simulink model "reorder_test"  (Simulink 8.0)
settings: Solver=ode45  StartTime=0.0  StopTime=1e5+1000  RelTol=1e-3
libraries: xbsIndex_r4 x486, casper_library_delays x4, xps_library x3
(part 1 of 3)
settings Model: Creator=davidm  LastModifiedBy=davidm

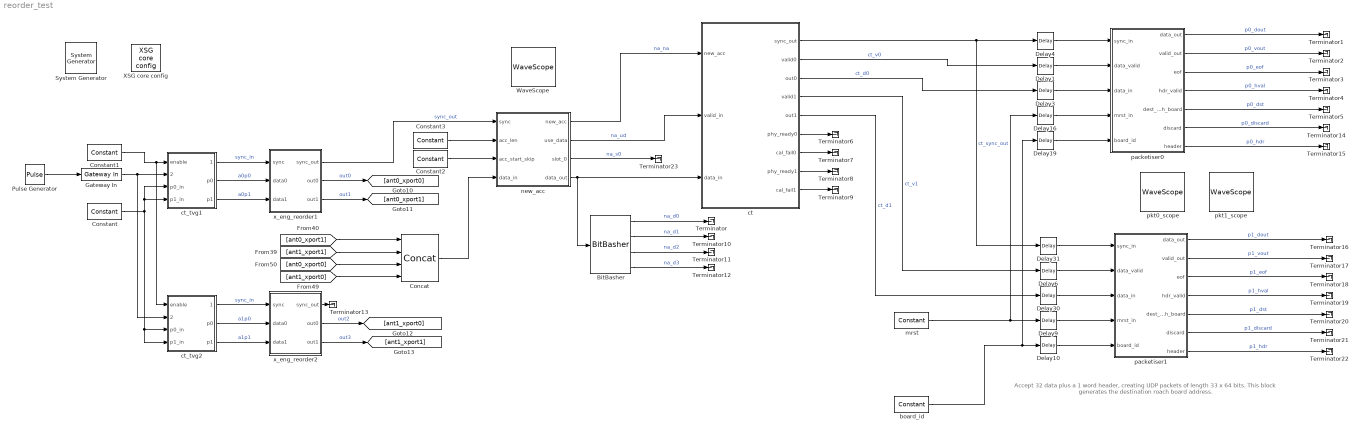
== system reorder_test ==
  note: Accept 32 data plus a 1 word header,
      | creating UDP packets of length 33 x 64 bits.
      | This block generates the destination roach board address.
  " System Generator" : xbsIndex_r4/ System Generator  Tag=genX  xilinxfamily=Kintex7  part=xc7k325t  speed=-3  package=fbg676  synthesis_tool=XST  clock_wrapper=Clock Enables  directory=./netlist  proj_type=Project Navigator  Synth_file=XST Defaults  Impl_file=ISE Defaults  testbench=off  simulink_period=1  sysclk_period=10  dcm_input_clock_period=10  incr_netlist=off  trim_vbits=Everywhere in SubSystem  dbl_ovrd=According to Block Masks  core_generation=According to Block Masks  run_coregen=off  deprecated_control=off  eval_field=0  block_type=sysgen
  BitBasher : xbsIndex_r4/BitBasher  bitexpr=|  display_expr=off  sr_1=1  arith_type1=Unsigned  bin_pt1=0  sr_2=2  arith_type2=Unsigned  bin_pt2=0  sr_3=3  arith_type3=Unsigned  bin_pt3=0  sr_4=4  arith_type4=Unsigned  bin_pt4=0  dbl_ovrd=off  block_type=bitbasher
      | <!DOCTYPE HTML PUBLIC "-//W3C//DTD HTML 4.0//EN" "http://www.w3.org/TR/REC-html40/strict.dtd">
      | <html><head><meta name="qrichtext" content="1" /><style type="text/css">
      | p, li { white-space: pre-wrap; }
      | </style></head><body style=" font-family:'Sans'; font-size:10pt; font-weight:400; font-style:normal;">
      | <p style=" margin-top:12px; margin-bottom:12px; margin-left:0px; margin-right:0px; -qt-block-indent:0; text-indent:0px;"><span style=" font-family:'MS Shell Dlg'; font-size:8pt;">o0={o[63:48]}<br />o1={o[47:32]}<br />o2={o[31:16]}<br />o3={o[15:0]}</span></p></body></html>
  Concat : xbsIndex_r4/Concat  num_inputs=4  dbl_ovrd=off  block_type=concat
  Constant : xbsIndex_r4/Constant  const=hex2dec('dada')  gui_display_data_type=Fixed-point  arith_type=Unsigned  n_bits=16  bin_pt=0  preci_type=Single  exp_width=8  frac_width=24  explicit_period=on  period=1  equ=P=C  opselect=C  inp2=PCIN>>17  opr=+  inp1=P  carry=CIN  dbl_ovrd=off  block_type=constant
  Constant1 : xbsIndex_r4/Constant  const=1  gui_display_data_type=Fixed-point  arith_type=Unsigned  n_bits=1  bin_pt=0  preci_type=Single  exp_width=8  frac_width=24  explicit_period=on  period=1  equ=P=C  opselect=C  inp2=PCIN>>17  opr=+  inp1=P  carry=CIN  dbl_ovrd=off  block_type=constant
  Constant2 : xbsIndex_r4/Constant  const=1  gui_display_data_type=Fixed-point  arith_type=Unsigned  n_bits=16  bin_pt=0  preci_type=Single  exp_width=8  frac_width=24  explicit_period=on  period=1  equ=P=C  opselect=C  inp2=PCIN>>17  opr=+  inp1=P  carry=CIN  dbl_ovrd=off  block_type=constant
  Constant3 : xbsIndex_r4/Constant  const=8  gui_display_data_type=Fixed-point  arith_type=Unsigned  n_bits=16  bin_pt=0  preci_type=Single  exp_width=8  frac_width=24  explicit_period=on  period=1  equ=P=C  opselect=C  inp2=PCIN>>17  opr=+  inp1=P  carry=CIN  dbl_ovrd=off  block_type=constant
  Delay{1,3..4,6,9..10,16,19,30..31} (10 alike) : xbsIndex_r4/Delay  rst=off  infoeditControl=Selection of Reset will increase slice count due to use of real FFs and instead of SRLs  en=off  latency=1  dbl_ovrd=off  reg_retiming=on  block_type=delay
      settings: xl_area=[0, 0, 0, 0, 0, 0, 0]
  Gateway In : xbsIndex_r4/Gateway In  gui_display_data_type=Boolean  arith_type=Boolean  n_bits=16  bin_pt=14  preci_type=Single  exp_width=8  frac_width=24  quantization="Round  (unbiased: +/- Inf)"  overflow=Saturate  period=1  dbl_ovrd=off  timing_constraint=None  locs_specified=off  LOCs={}  UseAsADC=off  ADCChannel='1'  inherit_from_input=off  hdl_port=on  block_type=gatewayin
  Pulse Generator : DiscretePulseGenerator  Period=1e9  PhaseDelay=2
  Terminator{,1..23} (24 alike) : Terminator
  WaveScope : xbsIndex_r4/WaveScope  block_type=wavescope
  XSG core config : xps_library/XSG core config  Tag=xps:xsg  hw_sys=ROACH2:sx475t  clk_src=sys_clk  ROACH_clk_src=sys_clk  ROACH2_clk_src=sys_clk  MKDIG_clk_src=sys_clk  clk_rate=100  sample_period=1  synthesis_tool=XST
  board_id : xbsIndex_r4/Constant  const=0  gui_display_data_type=Fixed-point  arith_type=Unsigned  n_bits=4  bin_pt=0  preci_type=Single  exp_width=8  frac_width=24  explicit_period=on  period=1  equ=P=C  opselect=C  inp2=PCIN>>17  opr=+  inp1=P  carry=CIN  dbl_ovrd=off  block_type=constant
  ct : Subsystem  mask{freq_chan=12, x_acc_len=3, bram_latency=2, ip_bits=16}
      mask prompts: freq_chan "No. of frequency channels (2 ^ ?)"; x_acc_len "X-eng Accumulation length (2^? samples):"; bram_latency "bram latency"; ip_bits "Input channel bitwidth"
  ct_tvg1 : Subsystem  mask{num_channels_bits=12, channel_bits=8, ant=0}
      mask prompts: num_channels_bits "Number of channels (2^?):"; channel_bits "Bits per channel:"; ant "Antenna # [0, 15]"
  ct_tvg2 : Subsystem  mask{num_channels_bits=12, channel_bits=8, ant=1}
      mask prompts: num_channels_bits "Number of channels (2^?):"; channel_bits "Bits per channel:"; ant "Antenna # [0, 15]"
  mrst : xbsIndex_r4/Constant  const=0  gui_display_data_type=Boolean  arith_type=Boolean  n_bits=4  bin_pt=0  preci_type=Single  exp_width=8  frac_width=24  explicit_period=on  period=1  equ=P=C  opselect=C  inp2=PCIN>>17  opr=+  inp1=P  carry=CIN  dbl_ovrd=off  block_type=constant
  new_acc : Subsystem
  packetiser0 : Subsystem  mask{payload_bits=1, n_x_board=2, freq_chan=12, n_boards=1, gbe_port=0}
      mask prompts: payload_bits "Payload length in 64bit words (2^?)"; n_x_board "Number of x-engines per ROACH board (2^?)"; freq_chan "Number of frequencies (2^?)"; n_boards "Number of  ROACH boards (2 ^ ?)"; gbe_port "Port # (0 or 1)"
      mask help: Package 32 bit data into 64 bits and identify data as coming from antenna 0 or 1
      mask init:
      | n_x = n_x_board - 1;
  packetiser1 : Subsystem  mask{payload_bits=1, n_x_board=2, freq_chan=12, n_boards=1, gbe_port=1}
      mask prompts: payload_bits "Payload length in 64bit words (2^?)"; n_x_board "Number of x-engines per ROACH board (2^?)"; freq_chan "Number of frequencies (2^?)"; n_boards "Number of  ROACH boards (2 ^ ?)"; gbe_port "Port # (0 or 1)"
      mask help: Package 32 bit data into 64 bits and identify data as coming from antenna 0 or 1
      mask init:
      | n_x = n_x_board - 1;
  pkt0_scope : xbsIndex_r4/WaveScope  block_type=wavescope
  pkt1_scope : xbsIndex_r4/WaveScope  block_type=wavescope
  x_eng_reorder1 : Subsystem  mask{freq_chan=12, num_data_bits=16, bram_latency=2, n_boards=1, n_x_board=2}
      mask prompts: freq_chan "Number of Frequency Channels (2 ^ ?)"; num_data_bits "Incomin data width in bits"; bram_latency "BRAM Latency"; n_boards "Number of ROACH boards (2 ^ ?)"; n_x_board "Number of X-engines per ROACH board (2 ^ ?)"
      mask help:
      | Reorders channels for transmission to X-engines in two stages.
      |
      | In the first stage, total of P channels on both inputs (P/2 on each input)
      | are reordered as follows:
      |
      | Input data0 has channels: 0, 2, 4, ..., P-2.
      | Input data1 has channels: 1, 3, 5, ..., P-1.
      | Then,
      | Output out0 has channels: 0, 1, 2, ..., P/2 -1.
      | Output out1 has channels: P/2, P/2 + 1, ..., P-1.
      |
      | Here P = 2 ^ (N - B),
      | where 2 ^ N = no. of total frequency channels
      | and 2 ^ B = total number of ROACH boards
      |
      | In the second stage, the channels on the each output are reordered in a way
      | that when presented to the 10 GbE port, they appear in the following order:
      | First channel to the first X-engine connected to the receiving 10gbE port of all ROACH boards.
      | First channel to the second X-engine connected to the receiving 10GbE port of all ROACH boards.
      | and so on.
      mask init:
      | n_x = n_x_board - 1;
  x_eng_reorder2 : Subsystem  mask{freq_chan=12, num_data_bits=16, bram_latency=2, n_boards=1, n_x_board=2}
      mask prompts: freq_chan "Number of Frequency Channels (2 ^ ?)"; num_data_bits "Incomin data width in bits"; bram_latency "BRAM Latency"; n_boards "Number of ROACH boards (2 ^ ?)"; n_x_board "Number of X-engines per ROACH board (2 ^ ?)"
      mask help:
      | Reorders channels for transmission to X-engines in two stages.
      |
      | In the first stage, total of P channels on both inputs (P/2 on each input)
      | are reordered as follows:
      |
      | Input data0 has channels: 0, 2, 4, ..., P-2.
      | Input data1 has channels: 1, 3, 5, ..., P-1.
      | Then,
      | Output out0 has channels: 0, 1, 2, ..., P/2 -1.
      | Output out1 has channels: P/2, P/2 + 1, ..., P-1.
      |
      | Here P = 2 ^ (N - B),
      | where 2 ^ N = no. of total frequency channels
      | and 2 ^ B = total number of ROACH boards
      |
      | In the second stage, the channels on the each output are reordered in a way
      | that when presented to the 10 GbE port, they appear in the following order:
      | First channel to the first X-engine connected to the receiving 10gbE port of all ROACH boards.
      | First channel to the second X-engine connected to the receiving 10GbE port of all ROACH boards.
      | and so on.
      mask init:
      | n_x = n_x_board - 1;
  wires:
  ct_tvg1/1(sync_out) -> x_eng_reorder1/1(sync)  "sync_in"
  ct_tvg1/2(p0) -> x_eng_reorder1/2(data0)  "a0p0"
  ct_tvg1/3(p1) -> x_eng_reorder1/3(data1)  "a0p1"
  Pulse Generator/1 -> Gateway In/1
  Gateway In/1 -> ct_tvg2/2(sync_in), ct_tvg1/2(sync_in)
  Constant/1 -> ct_tvg2/4(p1_in), ct_tvg2/3(p0_in), ct_tvg1/4(p1_in), ct_tvg1/3(p0_in)
  Constant1/1 -> ct_tvg2/1(enable), ct_tvg1/1(enable)
  x_eng_reorder1/1(sync_out) -> new_acc/1(sync)  "sync_out"
  x_eng_reorder1/2(out0) -> [ant0_xport0]  "out0"
  x_eng_reorder1/3(out1) -> [ant0_xport1]  "out1"
  Constant2/1 -> new_acc/3(acc_start_skip)
  Constant3/1 -> new_acc/2(acc_len)
  new_acc/1(new_acc) -> ct/1(new_acc)  "na_na"
  new_acc/2(use_data) -> ct/2(valid_in)  "na_ud"
  new_acc/4(data_out) -> BitBasher/1, ct/3(data_in)
  ct/1(sync_out) -> Delay4/1, Delay31/1  "ct_sync_out"
  ct/2(valid0) -> Delay1/1  "ct_v0"
  ct/3(out0) -> Delay3/1  "ct_d0"
  ct/4(valid1) -> Delay6/1  "ct_v1"
  ct/5(out1) -> Delay30/1  "ct_d1"
  ct/6(phy_ready0) -> Terminator6/1
  ct/7(cal_fail0) -> Terminator7/1
  ct/8(phy_ready1) -> Terminator8/1
  ct/9(cal_fail1) -> Terminator9/1
  ct_tvg2/1(sync_out) -> x_eng_reorder2/1(sync)  "sync_in"
  ct_tvg2/2(p0) -> x_eng_reorder2/2(data0)  "a1p0"
  ct_tvg2/3(p1) -> x_eng_reorder2/3(data1)  "a1p1"
  x_eng_reorder2/2(out0) -> [ant1_xport0]  "out2"
  x_eng_reorder2/3(out1) -> [ant1_xport1]  "out3"
  Concat/1 -> new_acc/4(data_in)
  BitBasher/1 -> Terminator/1  "na_d0"
  BitBasher/2 -> Terminator10/1  "na_d1"
  BitBasher/3 -> Terminator11/1  "na_d2"
  BitBasher/4 -> Terminator12/1  "na_d3"
  x_eng_reorder2/1(sync_out) -> Terminator13/1
  Delay4/1 -> packetiser0/1(sync_in)
  Delay1/1 -> packetiser0/2(data_valid)
  Delay3/1 -> packetiser0/3(data_in)
  Delay16/1 -> packetiser0/4(mrst_in)
  Delay19/1 -> packetiser0/5(board_id)
  Delay31/1 -> packetiser1/1(sync_in)
  Delay6/1 -> packetiser1/2(data_valid)
  Delay30/1 -> packetiser1/3(data_in)
  Delay9/1 -> packetiser1/4(mrst_in)
  Delay10/1 -> packetiser1/5(board_id)
  board_id/1 -> Delay19/1, Delay10/1
  mrst/1 -> Delay16/1, Delay9/1
  packetiser0/1(data_out) -> Terminator1/1  "p0_dout"
  packetiser0/2(valid_out) -> Terminator2/1  "p0_vout"
  packetiser0/3(eof) -> Terminator3/1  "p0_eof"
  packetiser0/4(hdr_valid) -> Terminator4/1  "p0_hval"
  packetiser0/5(dest_roach_board) -> Terminator5/1  "p0_dst"
  packetiser0/6(discard) -> Terminator14/1  "p0_discard"
  packetiser0/7(header) -> Terminator15/1  "p0_hdr"
  packetiser1/1(data_out) -> Terminator16/1  "p1_dout"
  packetiser1/2(valid_out) -> Terminator17/1  "p1_vout"
  packetiser1/3(eof) -> Terminator18/1  "p1_eof"
  packetiser1/4(hdr_valid) -> Terminator19/1  "p1_hval"
  packetiser1/5(dest_roach_board) -> Terminator20/1  "p1_dst"
  packetiser1/6(discard) -> Terminator21/1  "p1_discard"
  packetiser1/7(header) -> Terminator22/1  "p1_hdr"
  [ant0_xport1] -> Concat/1
  [ant1_xport1] -> Concat/2
  [ant0_xport0] -> Concat/3
  [ant1_xport0] -> Concat/4
  new_acc/3(slot_0) -> Terminator23/1  "na_s0"

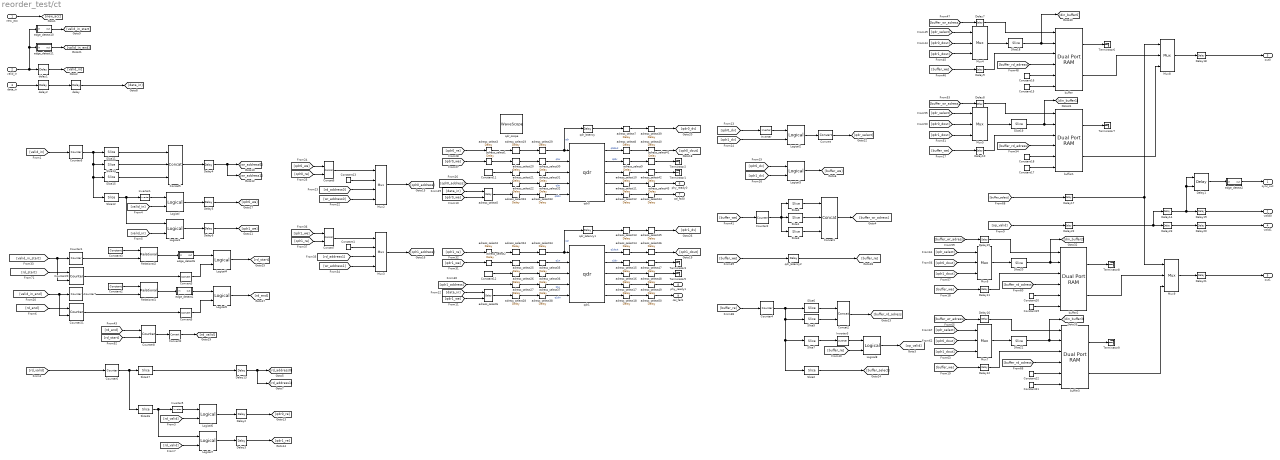
== system reorder_test/ct ==
  new_acc : Inport
  valid_in : Inport  Port=2
  data_in : Inport  Port=3
  Concat1 : xbsIndex_r4/Concat  num_inputs=3  dbl_ovrd=off  block_type=concat
  Concat2 : xbsIndex_r4/Concat  num_inputs=2  dbl_ovrd=off  block_type=concat
  Concat5 : xbsIndex_r4/Concat  num_inputs=3  dbl_ovrd=off  block_type=concat
  Concat6 : xbsIndex_r4/Concat  num_inputs=2  dbl_ovrd=off  block_type=concat
  Concat7 : xbsIndex_r4/Concat  num_inputs=2  dbl_ovrd=off  block_type=concat
  Constant1 : xbsIndex_r4/Constant  const=0  gui_display_data_type=Fixed-point  arith_type=Unsigned  n_bits=freq_chan + x_acc_len - 1  bin_pt=0  preci_type=Single  exp_width=8  frac_width=24  explicit_period=on  period=1  equ=P=C  opselect=C  inp2=PCIN>>17  opr=+  inp1=P  carry=CIN  dbl_ovrd=off  block_type=constant
      settings: block_version=11.4
  Constant11 : xbsIndex_r4/Constant  const=255  gui_display_data_type=Fixed-point  arith_type=Unsigned  n_bits=8  bin_pt=0  preci_type=Single  exp_width=8  frac_width=24  explicit_period=on  period=1  equ=P=C  opselect=C  inp2=PCIN>>17  opr=+  inp1=P  carry=CIN  dbl_ovrd=off  block_type=constant
  Constant12 : xbsIndex_r4/Constant  const=255  gui_display_data_type=Fixed-point  arith_type=Unsigned  n_bits=8  bin_pt=0  preci_type=Single  exp_width=8  frac_width=24  explicit_period=on  period=1  equ=P=C  opselect=C  inp2=PCIN>>17  opr=+  inp1=P  carry=CIN  dbl_ovrd=off  block_type=constant
  Constant13 : xbsIndex_r4/Constant  const=0  gui_display_data_type=Fixed-point  arith_type=Unsigned  n_bits=freq_chan + x_acc_len - 1  bin_pt=0  preci_type=Single  exp_width=8  frac_width=24  explicit_period=on  period=1  equ=P=C  opselect=C  inp2=PCIN>>17  opr=+  inp1=P  carry=CIN  dbl_ovrd=off  block_type=constant
      settings: block_version=11.4
  Constant{15,17,19,21} (4 alike) : xbsIndex_r4/Constant  const=0  gui_display_data_type=Fixed-point  arith_type=Boolean  n_bits=16  bin_pt=14  preci_type=Single  exp_width=8  frac_width=24  explicit_period=on  period=1  equ=P=C  opselect=C  inp2=PCIN>>17  opr=+  inp1=P  carry=CIN  dbl_ovrd=off  block_type=constant
      settings: block_version=11.4
  Constant{16,18,20,22} (4 alike) : xbsIndex_r4/Constant  const=0  gui_display_data_type=Fixed-point  arith_type=Unsigned  n_bits=64  bin_pt=0  preci_type=Single  exp_width=8  frac_width=24  explicit_period=on  period=1  equ=P=C  opselect=C  inp2=PCIN>>17  opr=+  inp1=P  carry=CIN  dbl_ovrd=off  block_type=constant
      settings: block_version=11.4
  Constant2 : xbsIndex_r4/Constant  const=2 ^ (freq_chan + x_acc_len - 1) - 3  gui_display_data_type=Fixed-point  arith_type=Unsigned  n_bits=freq_chan + x_acc_len - 1  bin_pt=0  preci_type=Single  exp_width=8  frac_width=24  explicit_period=on  period=1  equ=P=C  opselect=C  inp2=PCIN>>17  opr=+  inp1=P  carry=CIN  dbl_ovrd=off  block_type=constant
      settings: block_version=11.4
  Constant3 : xbsIndex_r4/Constant  const=2 ^ (freq_chan + x_acc_len - 1) - 3  gui_display_data_type=Fixed-point  arith_type=Unsigned  n_bits=freq_chan + x_acc_len - 1  bin_pt=0  preci_type=Single  exp_width=8  frac_width=24  explicit_period=on  period=1  equ=P=C  opselect=C  inp2=PCIN>>17  opr=+  inp1=P  carry=CIN  dbl_ovrd=off  block_type=constant
      settings: block_version=11.4
  Convert : xbsIndex_r4/Convert  gui_display_data_type=Fixed-point  arith_type=Unsigned  n_bits=1  bin_pt=0  float_type=Single  exp_bits=8  fraction_bits=24  quantization=Truncate  overflow=Wrap  en=off  latency=0  dbl_ovrd=off  pipeline=off  block_type=convert
      settings: block_version=11.4
  Convert2 : xbsIndex_r4/Convert  gui_display_data_type=Fixed-point  arith_type=Boolean  n_bits=16  bin_pt=14  float_type=Single  exp_bits=8  fraction_bits=24  quantization=Truncate  overflow=Wrap  en=off  latency=0  dbl_ovrd=off  pipeline=off  block_type=convert
      settings: block_version=11.4
  Convert3 : xbsIndex_r4/Convert  gui_display_data_type=Fixed-point  arith_type=Boolean  n_bits=16  bin_pt=14  float_type=Single  exp_bits=8  fraction_bits=24  quantization=Truncate  overflow=Wrap  en=off  latency=0  dbl_ovrd=off  pipeline=off  block_type=convert
      settings: block_version=11.4
  Convert5 : xbsIndex_r4/Convert  gui_display_data_type=Fixed-point  arith_type=Boolean  n_bits=16  bin_pt=14  float_type=Single  exp_bits=8  fraction_bits=24  quantization=Truncate  overflow=Wrap  en=off  latency=0  dbl_ovrd=off  pipeline=off  block_type=convert
      settings: block_version=11.4
  Counter1 : xbsIndex_r4/Counter  cnt_type=Free Running  cnt_to=10  operation=Up  start_count=0  cnt_by_val=1  arith_type=Unsigned  n_bits=freq_chan + x_acc_len - 1  bin_pt=0  load_pin=off  rst=on  en=off  explicit_period=off  period=1  dbl_ovrd=off  use_behavioral_HDL=off  implementation=Fabric  block_type=counter
      settings: block_version=11.4
  Counter2 : xbsIndex_r4/Counter  cnt_type=Free Running  cnt_to=10  operation=Up  start_count=0  cnt_by_val=1  arith_type=Unsigned  n_bits=x_acc_len + 2  bin_pt=0  load_pin=off  rst=off  en=on  explicit_period=off  period=1  dbl_ovrd=off  use_behavioral_HDL=off  implementation=Fabric  block_type=counter
      settings: block_version=11.4
  Counter20 : xbsIndex_r4/Counter  cnt_type=Free Running  cnt_to=10  operation=Up  start_count=0  cnt_by_val=1  arith_type=Unsigned  n_bits=1  bin_pt=0  load_pin=off  rst=on  en=on  explicit_period=off  period=1  dbl_ovrd=off  use_behavioral_HDL=off  implementation=Fabric  block_type=counter
      settings: block_version=11.4
  Counter21 : xbsIndex_r4/Counter  cnt_type=Free Running  cnt_to=10  operation=Up  start_count=0  cnt_by_val=1  arith_type=Unsigned  n_bits=1  bin_pt=0  load_pin=off  rst=on  en=on  explicit_period=off  period=1  dbl_ovrd=off  use_behavioral_HDL=off  implementation=Fabric  block_type=counter
      settings: block_version=11.4
  Counter4 : xbsIndex_r4/Counter  cnt_type=Free Running  cnt_to=10  operation=Up  start_count=0  cnt_by_val=1  arith_type=Unsigned  n_bits=x_acc_len + 2  bin_pt=0  load_pin=off  rst=off  en=on  explicit_period=off  period=1  dbl_ovrd=off  use_behavioral_HDL=off  implementation=Fabric  block_type=counter
      settings: block_version=11.4
  Counter5 : xbsIndex_r4/Counter  cnt_type=Free Running  cnt_to=10  operation=Up  start_count=0  cnt_by_val=1  arith_type=Unsigned  n_bits=freq_chan + x_acc_len  bin_pt=0  load_pin=off  rst=off  en=on  explicit_period=off  period=1  dbl_ovrd=off  use_behavioral_HDL=off  implementation=Fabric  block_type=counter
      settings: block_version=11.4
  Counter6 : xbsIndex_r4/Counter  cnt_type=Free Running  cnt_to=10  operation=Up  start_count=0  cnt_by_val=1  arith_type=Unsigned  n_bits=freq_chan + x_acc_len  bin_pt=0  load_pin=off  rst=off  en=on  explicit_period=off  period=1  dbl_ovrd=off  use_behavioral_HDL=off  implementation=Fabric  block_type=counter
      settings: block_version=11.4
  Counter7 : xbsIndex_r4/Counter  cnt_type=Free Running  cnt_to=10  operation=Up  start_count=0  cnt_by_val=1  arith_type=Unsigned  n_bits=freq_chan + x_acc_len - 1  bin_pt=0  load_pin=off  rst=on  en=off  explicit_period=off  period=1  dbl_ovrd=off  use_behavioral_HDL=off  implementation=Fabric  block_type=counter
      settings: block_version=11.4
  Counter8 : xbsIndex_r4/Counter  cnt_type=Free Running  cnt_to=10  operation=Up  start_count=0  cnt_by_val=1  arith_type=Unsigned  n_bits=1  bin_pt=0  load_pin=off  rst=on  en=on  explicit_period=off  period=1  dbl_ovrd=off  use_behavioral_HDL=off  implementation=Fabric  block_type=counter
      settings: block_version=11.4
  Delay1 : xbsIndex_r4/Delay  rst=off  infoeditControl=Selection of Reset will increase slice count due to use of real FFs and instead of SRLs  en=on  latency=1  dbl_ovrd=off  reg_retiming=on  block_type=delay
      settings: block_version=11.4
  Delay{2..16,23} (16 alike) : xbsIndex_r4/Delay  rst=off  infoeditControl=Selection of Reset will increase slice count due to use of real FFs and instead of SRLs  en=off  latency=1  dbl_ovrd=off  reg_retiming=on  block_type=delay
      settings: block_version=11.4
  Delay17 : xbsIndex_r4/Delay  rst=off  infoeditControl=Selection of Reset will increase slice count due to use of real FFs and instead of SRLs  en=off  latency=bram_latency  dbl_ovrd=off  reg_retiming=on  block_type=delay
      settings: block_version=11.4
  Delay{18..21} (4 alike) : xbsIndex_r4/Delay  rst=off  infoeditControl=Selection of Reset will increase slice count due to use of real FFs and instead of SRLs  en=off  latency=2  dbl_ovrd=off  reg_retiming=on  block_type=delay
      settings: block_version=11.4
  Delay22 : xbsIndex_r4/Delay  rst=off  infoeditControl=Selection of Reset will increase slice count due to use of real FFs and instead of SRLs  en=off  latency=bram_latency  dbl_ovrd=off  reg_retiming=on  block_type=delay
      settings: block_version=11.4
  Inverter{,1,3,5} (4 alike) : xbsIndex_r4/Inverter  en=off  latency=0  dbl_ovrd=off  block_type=inv
      settings: block_version=11.4
  Logical{,1..2,4..8} (8 alike) : xbsIndex_r4/Logical  logical_function=AND  inputs=2  en=off  latency=0  precision=Full  arith_type=Unsigned  n_bits=16  bin_pt=0  align_bp=on  dbl_ovrd=off  block_type=logical
      settings: block_version=11.4
  Logical3 : xbsIndex_r4/Logical  logical_function=XOR  inputs=2  en=off  latency=0  precision=Full  arith_type=Unsigned  n_bits=16  bin_pt=0  align_bp=on  dbl_ovrd=off  block_type=logical
      settings: block_version=11.4
  Mux2 : xbsIndex_r4/Mux  inputs=3  en=off  latency=1  precision=Full  arith_type=Unsigned  n_bits=16  bin_pt=14  quantization=Truncate  overflow=Wrap  dbl_ovrd=off  block_type=mux
      settings: block_version=11.4
  Mux3 : xbsIndex_r4/Mux  inputs=3  en=off  latency=1  precision=Full  arith_type=Unsigned  n_bits=16  bin_pt=14  quantization=Truncate  overflow=Wrap  dbl_ovrd=off  block_type=mux
      settings: block_version=11.4
  Mux{4..9} (6 alike) : xbsIndex_r4/Mux  inputs=2  en=off  latency=1  precision=Full  arith_type=Unsigned  n_bits=16  bin_pt=14  quantization=Truncate  overflow=Wrap  dbl_ovrd=off  block_type=mux
      settings: block_version=11.4
  Relational1 : xbsIndex_r4/Relational  mode=a=b  en=off  latency=1  dbl_ovrd=off  block_type=relational
  Relational2 : xbsIndex_r4/Relational  mode=a=b  en=off  latency=1  dbl_ovrd=off  block_type=relational
  Slice1 : xbsIndex_r4/Slice  nbits=1  boolean_output=off  mode=Lower Bit Location + Width  bit1=0  base1=MSB of Input  bit0=0  base0=LSB of Input  dbl_ovrd=off  block_type=slice
      settings: block_version=10.1.3
  Slice11 : xbsIndex_r4/Slice  nbits=1  boolean_output=off  mode=Upper Bit Location + Width  bit1=0  base1=MSB of Input  bit0=1  base0=LSB of Input  dbl_ovrd=off  block_type=slice
      settings: block_version=10.1.3
  Slice12 : xbsIndex_r4/Slice  nbits=1  boolean_output=on  mode=Lower Bit Location + Width  bit1=0  base1=MSB of Input  bit0=0  base0=LSB of Input  dbl_ovrd=off  block_type=slice
      settings: block_version=10.1.3
  Slice14 : xbsIndex_r4/Slice  nbits=freq_chan - 2  boolean_output=off  mode=Lower Bit Location + Width  bit1=0  base1=MSB of Input  bit0=1  base0=LSB of Input  dbl_ovrd=off  block_type=slice
      settings: block_version=10.1.3
  Slice15 : xbsIndex_r4/Slice  nbits=x_acc_len  boolean_output=off  mode=Lower Bit Location + Width  bit1=0  base1=MSB of Input  bit0=freq_chan - 1  base0=LSB of Input  dbl_ovrd=off  block_type=slice
      settings: block_version=10.1.3
  Slice16 : xbsIndex_r4/Slice  nbits=1  boolean_output=on  mode=Lower Bit Location + Width  bit1=0  base1=MSB of Input  bit0=0  base0=LSB of Input  dbl_ovrd=off  block_type=slice
      settings: block_version=10.1.3
  Slice17 : xbsIndex_r4/Slice  nbits=freq_chan + x_acc_len - 1  boolean_output=off  mode=Lower Bit Location + Width  bit1=0  base1=MSB of Input  bit0=1  base0=LSB of Input  dbl_ovrd=off  block_type=slice
      settings: block_version=10.1.3
  Slice18 : xbsIndex_r4/Slice  nbits=ip_bits  boolean_output=off  mode=Lower Bit Location + Width  bit1=0  base1=MSB of Input  bit0=ip_bits * 3  base0=LSB of Input  dbl_ovrd=off  block_type=slice
      settings: block_version=10.1.3
  Slice19 : xbsIndex_r4/Slice  nbits=ip_bits  boolean_output=off  mode=Lower Bit Location + Width  bit1=0  base1=MSB of Input  bit0=ip_bits * 2  base0=LSB of Input  dbl_ovrd=off  block_type=slice
      settings: block_version=10.1.3
  Slice2 : xbsIndex_r4/Slice  nbits=1  boolean_output=off  mode=Lower Bit Location + Width  bit1=0  base1=MSB of Input  bit0=x_acc_len - 1  base0=LSB of Input  dbl_ovrd=off  block_type=slice
      settings: block_version=10.1.3
  Slice20 : xbsIndex_r4/Slice  nbits=ip_bits  boolean_output=off  mode=Lower Bit Location + Width  bit1=0  base1=MSB of Input  bit0=ip_bits  base0=LSB of Input  dbl_ovrd=off  block_type=slice
      settings: block_version=10.1.3
  Slice21 : xbsIndex_r4/Slice  nbits=ip_bits  boolean_output=off  mode=Lower Bit Location + Width  bit1=0  base1=MSB of Input  bit0=0  base0=LSB of Input  dbl_ovrd=off  block_type=slice
      settings: block_version=10.1.3
  Slice3 : xbsIndex_r4/Slice  nbits=x_acc_len  boolean_output=off  mode=Lower Bit Location + Width  bit1=0  base1=MSB of Input  bit0=1  base0=LSB of Input  dbl_ovrd=off  block_type=slice
      settings: block_version=10.1.3
  Slice4 : xbsIndex_r4/Slice  nbits=1  boolean_output=on  mode=Upper Bit Location + Width  bit1=0  base1=MSB of Input  bit0=0  base0=LSB of Input  dbl_ovrd=off  block_type=slice
      settings: block_version=10.1.3
  Slice5 : xbsIndex_r4/Slice  nbits=x_acc_len - 2  boolean_output=off  mode=Lower Bit Location + Width  bit1=0  base1=MSB of Input  bit0=0  base0=LSB of Input  dbl_ovrd=off  block_type=slice
      settings: block_version=10.1.3
  Slice6 : xbsIndex_r4/Slice  nbits=2  boolean_output=off  mode=Upper Bit Location + Width  bit1=0  base1=MSB of Input  bit0=0  base0=LSB of Input  dbl_ovrd=off  block_type=slice
      settings: block_version=10.1.3
  Slice7 : xbsIndex_r4/Slice  nbits=1  boolean_output=on  mode=Lower Bit Location + Width  bit1=0  base1=MSB of Input  bit0=x_acc_len - 2  base0=LSB of Input  dbl_ovrd=off  block_type=slice
      settings: block_version=10.1.3
  Terminator{1..3,5..9} (8 alike) : Terminator
  adress_select{1..4,7..50} (48 alike) : xbsIndex_r4/Delay  rst=off  infoeditControl=Selection of Reset will increase slice count due to use of real FFs and instead of SRLs  en=off  latency=1  dbl_ovrd=off  reg_retiming=on  block_type=delay
      settings: block_version=11.4
  adress_select5 : xbsIndex_r4/Delay  rst=off  infoeditControl=Selection of Reset will increase slice count due to use of real FFs and instead of SRLs  en=on  latency=1  dbl_ovrd=off  reg_retiming=on  block_type=delay
      settings: block_version=11.4
  adress_select6 : xbsIndex_r4/Delay  rst=off  infoeditControl=Selection of Reset will increase slice count due to use of real FFs and instead of SRLs  en=on  latency=1  dbl_ovrd=off  reg_retiming=on  block_type=delay
      settings: block_version=11.4
  buffer{,1..3} (4 alike) : xbsIndex_r4/Dual Port RAM  depth=2 ^ (x_acc_len + 2)  initVector=0  distributed_mem=Block RAM  init_a=0  init_b=0  rst_a=off  rst_b=off  en_a=off  en_b=off  latency=bram_latency  write_mode_A=Read Before Write  write_mode_B=Read Before Write  dbl_ovrd=off  optimize=Area  block_type=dpram
      settings: block_version=11.4
  delay : xbsIndex_r4/Delay  rst=off  infoeditControl=Selection of Reset will increase slice count due to use of real FFs and instead of SRLs  en=off  latency=1  dbl_ovrd=off  reg_retiming=on  block_type=delay
      settings: block_version=11.4
  delay1 : xbsIndex_r4/Delay  rst=off  infoeditControl=Selection of Reset will increase slice count due to use of real FFs and instead of SRLs  en=off  latency=1  dbl_ovrd=off  reg_retiming=on  block_type=delay
      settings: block_version=11.4
  delay2 : xbsIndex_r4/Delay  rst=off  infoeditControl=Selection of Reset will increase slice count due to use of real FFs and instead of SRLs  en=off  latency=1  dbl_ovrd=off  reg_retiming=on  block_type=delay
      settings: block_version=11.4
  edge_detect1 : Subsystem  AncestorBlock=casper_library_misc/edge_detect  mask(edge_detect){edge=Rising, polarity=Active High, x_in=[0 0.08 0.08 0.16 0.16 0.24 0.24 0.32 0.32 0.4], y_in=[-1 -1  1  1  1  1  1  1  1  1], x_out=[0.6 0.68 0.68 0.76 0.76 0.84 0.84 0.92 0.92 1], y_out=[-1 -1  1  1 -1 -1 -1 -1 -1 -1]}
      mask prompts: edge "Edge Type"; polarity "Output Polarity"; x_in "Input X Positions"; y_in "Input Y Positions"; x_out "Output X Positions"; y_out "Output Y Positions"
      mask help: Output is active for one-cycle after each edge of the specified type (i.e. rising, falling or both).
      mask init:
      | edge_detect_init(gcb,...
      |     'edge',edge,...
      |     'polarity',polarity,...
      |     'x_in',x_in,...
      |     'x_out',x_out,...
      |     'y_in',y_in,...
      |     'y_out',y_out);
      | 
      | x_in_num=str2num(getfield(getfield(get_param(gcb,'UserData'),'parameters'),'x_in'));
      | x_out_num=str2num(getfield(getfield(get_param(gcb,'UserData'),'parameters'),'x_out'));
      | y_in_num=str2num(getfield(getfield(get_param(gcb,'UserData'),'parameters'),'y_in'));
      | y_out_num=str2num(getfield(getfield(get_param(gcb,'UserData'),'parameters'),'y_out'));
      settings: AttributesFormatString=|
      | rising edges
      | active high
      mask Help: Output is active for one-cycle after each edge of the specified type (i.e. rising, falling, or both).  Latency is zero.
      mask TypeOptions edge: Rising | Falling | Both
      mask TypeOptions polarity: Active High | Active Low
      mask Display:
      | plot(x_in_num,0.5+y_in_num*0.2);
      | plot(x_out_num,0.5+y_out_num*0.2);
  edge_detect10 : Subsystem  AncestorBlock=casper_library_misc/edge_detect  mask(edge_detect){edge=Rising, polarity=Active High, x_in=[0 0.08 0.08 0.16 0.16 0.24 0.24 0.32 0.32 0.4], y_in=[-1 -1  1  1  1  1  1  1  1  1], x_out=[0.6 0.68 0.68 0.76 0.76 0.84 0.84 0.92 0.92 1], y_out=[-1 -1  1  1 -1 -1 -1 -1 -1 -1]}
      mask prompts: edge "Edge Type"; polarity "Output Polarity"; x_in "Input X Positions"; y_in "Input Y Positions"; x_out "Output X Positions"; y_out "Output Y Positions"
      mask help: Output is active for one-cycle after each edge of the specified type (i.e. rising, falling or both).
      mask init: same as reorder_test/ct/edge_detect1
      settings: AttributesFormatString=|
      | rising edges
      | active high
      mask Help: Output is active for one-cycle after each edge of the specified type (i.e. rising, falling, or both).  Latency is zero.
      mask TypeOptions edge: Rising | Falling | Both
      mask TypeOptions polarity: Active High | Active Low
      mask Display:
      | plot(x_in_num,0.5+y_in_num*0.2);
      | plot(x_out_num,0.5+y_out_num*0.2);
  edge_detect11 : Subsystem  AncestorBlock=casper_library_misc/edge_detect  mask(edge_detect){edge=Falling, polarity=Active High, x_in=[0 0.08 0.08 0.16 0.16 0.24 0.24 0.32 0.32 0.4], y_in=[1  1 -1 -1 -1 -1 -1 -1 -1 -1], x_out=[0.6 0.68 0.68 0.76 0.76 0.84 0.84 0.92 0.92 1], y_out=[-1 -1  1  1 -1 -1 -1 -1 -1 -1]}
      mask prompts: edge "Edge Type"; polarity "Output Polarity"; x_in "Input X Positions"; y_in "Input Y Positions"; x_out "Output X Positions"; y_out "Output Y Positions"
      mask help: Output is active for one-cycle after each edge of the specified type (i.e. rising, falling or both).
      mask init: same as reorder_test/ct/edge_detect1
      settings: AttributesFormatString=|
      | falling edges
      | active high
      mask Help: Output is active for one-cycle after each edge of the specified type (i.e. rising, falling, or both).  Latency is zero.
      mask TypeOptions edge: Rising | Falling | Both
      mask TypeOptions polarity: Active High | Active Low
      mask Display:
      | plot(x_in_num,0.5+y_in_num*0.2);
      | plot(x_out_num,0.5+y_out_num*0.2);
  edge_detect2 : Subsystem  AncestorBlock=casper_library_misc/edge_detect  mask(edge_detect){edge=Rising, polarity=Active High, x_in=[0 0.08 0.08 0.16 0.16 0.24 0.24 0.32 0.32 0.4], y_in=[-1 -1  1  1  1  1  1  1  1  1], x_out=[0.6 0.68 0.68 0.76 0.76 0.84 0.84 0.92 0.92 1], y_out=[-1 -1  1  1 -1 -1 -1 -1 -1 -1]}
      mask prompts: edge "Edge Type"; polarity "Output Polarity"; x_in "Input X Positions"; y_in "Input Y Positions"; x_out "Output X Positions"; y_out "Output Y Positions"
      mask help: Output is active for one-cycle after each edge of the specified type (i.e. rising, falling or both).
      mask init: same as reorder_test/ct/edge_detect1
      settings: AttributesFormatString=|
      | rising edges
      | active high
      mask Help: Output is active for one-cycle after each edge of the specified type (i.e. rising, falling, or both).  Latency is zero.
      mask TypeOptions edge: Rising | Falling | Both
      mask TypeOptions polarity: Active High | Active Low
      mask Display:
      | plot(x_in_num,0.5+y_in_num*0.2);
      | plot(x_out_num,0.5+y_out_num*0.2);
  edge_detect6 : Subsystem  AncestorBlock=casper_library_misc/edge_detect  mask(edge_detect){edge=Rising, polarity=Active High, x_in=[0 0.08 0.08 0.16 0.16 0.24 0.24 0.32 0.32 0.4], y_in=[-1 -1  1  1  1  1  1  1  1  1], x_out=[0.6 0.68 0.68 0.76 0.76 0.84 0.84 0.92 0.92 1], y_out=[-1 -1  1  1 -1 -1 -1 -1 -1 -1]}
      mask prompts: edge "Edge Type"; polarity "Output Polarity"; x_in "Input X Positions"; y_in "Input Y Positions"; x_out "Output X Positions"; y_out "Output Y Positions"
      mask help: Output is active for one-cycle after each edge of the specified type (i.e. rising, falling or both).
      mask init: same as reorder_test/ct/edge_detect1
      settings: AttributesFormatString=|
      | rising edges
      | active high
      mask Help: Output is active for one-cycle after each edge of the specified type (i.e. rising, falling, or both).  Latency is zero.
      mask TypeOptions edge: Rising | Falling | Both
      mask TypeOptions polarity: Active High | Active Low
      mask Display:
      | plot(x_in_num,0.5+y_in_num*0.2);
      | plot(x_out_num,0.5+y_out_num*0.2);
  qdr0 : xps_library/qdr  Tag=xps:qdr  which_qdr=qdr0  qdr_awidth=freq_chan + x_acc_len - 1  use_sniffer=on
      link override convert_be: n_bits=8
      link override convert_data_in: n_bits=72
      link override convert_data_in1: n_bits=72
      link override extract_parity: bitexpr=b = {a[71:0]}  arith_type1=Unsigned  arith_type2=Unsigned  arith_type3=Unsigned  arith_type4=Unsigned
      link override insert_parity: bitexpr=b = {a[71:0]}  arith_type1=Unsigned  arith_type2=Unsigned  arith_type3=Unsigned  arith_type4=Unsigned
      link override qdr_sim_model/sim_data_in: n_bits=72
      link override reorder_test_ct_qdr0_data_out: n_bits=72
  qdr1 : xps_library/qdr  Tag=xps:qdr  which_qdr=qdr1  qdr_awidth=freq_chan + x_acc_len - 1  use_sniffer=on
      link override convert_be: n_bits=8
      link override convert_data_in: n_bits=72
      link override convert_data_in1: n_bits=72
      link override extract_parity: bitexpr=b = {a[71:0]}  arith_type1=Unsigned  arith_type2=Unsigned  arith_type3=Unsigned  arith_type4=Unsigned
      link override insert_parity: bitexpr=b = {a[71:0]}  arith_type1=Unsigned  arith_type2=Unsigned  arith_type3=Unsigned  arith_type4=Unsigned
      link override qdr_sim_model/sim_data_in: n_bits=72
      link override reorder_test_ct_qdr1_data_out: n_bits=72
  qdr_latency : xbsIndex_r4/Delay  rst=off  infoeditControl=Selection of Reset will increase slice count due to use of real FFs and instead of SRLs  en=off  latency=10  dbl_ovrd=off  reg_retiming=on  block_type=delay
      settings: block_version=11.4
  qdr_latency1 : xbsIndex_r4/Delay  rst=off  infoeditControl=Selection of Reset will increase slice count due to use of real FFs and instead of SRLs  en=off  latency=10  dbl_ovrd=off  reg_retiming=on  block_type=delay
      settings: block_version=11.4
  qdr_latency2 : xbsIndex_r4/Delay  rst=off  infoeditControl=Selection of Reset will increase slice count due to use of real FFs and instead of SRLs  en=off  latency=2 ^ (x_acc_len + 1)  dbl_ovrd=off  reg_retiming=on  block_type=delay
      settings: block_version=11.4
  qdr_scope : xbsIndex_r4/WaveScope  block_type=wavescope
  sync_out : Outport
  valid0 : Outport  Port=2
  out0 : Outport  Port=3
  valid1 : Outport  Port=4
  out1 : Outport  Port=5
  phy_ready0 : Outport  Port=6
  cal_fail0 : Outport  Port=7
  phy_ready1 : Outport  Port=8
  cal_fail1 : Outport  Port=9
  wires:
  data_in/1 -> delay2/1
  new_acc/1 -> [new_acc]
  Counter5/1 -> Slice11/1, Slice14/1, Slice15/1, Slice12/1
  Slice11/1 -> Concat5/1
  Slice14/1 -> Concat5/2
  Slice15/1 -> Concat5/3
  Concat5/1 -> Delay4/1
  Slice12/1 -> Logical1/1, Inverter1/1
  Logical/1 -> Delay5/1
  Inverter1/1 -> Logical/1
  Delay4/1 -> [wr_address0], [wr_address1]
  Delay5/1 -> [qdr0_we]
  Logical1/1 -> Delay6/1
  Delay6/1 -> [qdr1_we]
  Constant11/1 -> adress_select21/1
  [qdr0_we] -> Concat6/1
  [qdr0_re] -> Concat6/2
  Concat6/1 -> Mux2/1
  Constant13/1 -> Mux2/2
  [rd_address0] -> Mux2/3
  [wr_address0] -> Mux2/4
  Mux2/1 -> [qdr0_address]
  [qdr0_address] -> adress_select22/1
  [qdr0_re] -> adress_select3/1
  [qdr0_we] -> adress_select1/1
  [data_in] -> adress_select5/1
  Constant12/1 -> adress_select26/1
  [qdr1_address] -> adress_select27/1
  [qdr1_re] -> adress_select4/1
  [qdr1_we] -> adress_select2/1
  [qdr1_we] -> Concat7/1
  [qdr1_re] -> Concat7/2
  Concat7/1 -> Mux3/1
  Constant1/1 -> Mux3/2
  [rd_address1] -> Mux3/3
  [wr_address1] -> Mux3/4
  Mux3/1 -> [qdr1_address]
  Constant16/1 -> buffer/5
  Constant15/1 -> buffer/6
  qdr0/1 -> adress_select8/1  "q0dout"
  qdr1/1 -> adress_select14/1  "q1dout"
  Mux4/1 -> Slice18/1
  [qdr0_dout] -> Mux4/2
  [qdr1_dout] -> Mux4/3
  [buffer_we] -> Delay9/1
  Delay9/1 -> buffer/3
  [buffer_rd_adress] -> buffer/4
  [qdr_select] -> Mux4/1
  Constant18/1 -> buffer1/5
  Constant17/1 -> buffer1/6
  Mux5/1 -> Slice19/1
  [qdr0_dout] -> Mux5/2
  [qdr1_dout] -> Mux5/3
  Slice19/1 -> buffer1/2, [din_buffer1]
  [buffer_we] -> Delay10/1
  Delay10/1 -> buffer1/3
  [buffer_rd_adress] -> buffer1/4
  [qdr_select] -> Mux5/1
  Constant20/1 -> buffer2/5
  Constant19/1 -> buffer2/6
  Mux6/1 -> Slice20/1
  [qdr0_dout] -> Mux6/2
  [qdr1_dout] -> Mux6/3
  Slice20/1 -> buffer2/2, [din_buffer2]
  [buffer_we] -> Delay11/1
  Delay11/1 -> buffer2/3
  [buffer_rd_adress] -> buffer2/4
  [qdr_select] -> Mux6/1
  Constant22/1 -> buffer3/5
  Constant21/1 -> buffer3/6
  Mux7/1 -> Slice21/1
  [qdr0_dout] -> Mux7/2
  [qdr1_dout] -> Mux7/3
  Slice21/1 -> buffer3/2, [din_buffer3]
  [buffer_we] -> Delay12/1
  Delay12/1 -> buffer3/3
  [buffer_rd_adress] -> buffer3/4
  [qdr_select] -> Mux7/1
  buffer/1 -> Terminator6/1
  buffer1/1 -> Terminator7/1
  buffer2/1 -> Terminator8/1
  buffer3/1 -> Terminator9/1
  buffer/2 -> Mux8/2
  buffer1/2 -> Mux8/3
  Mux8/1 -> Delay18/1
  buffer2/2 -> Mux9/2
  buffer3/2 -> Mux9/3
  Mux9/1 -> Delay21/1
  qdr0/3 -> adress_select10/1
  qdr1/3 -> adress_select16/1
  qdr0/4 -> adress_select11/1
  qdr0/5 -> adress_select12/1
  qdr1/4 -> adress_select17/1
  qdr1/5 -> adress_select18/1
  adress_select1/1 -> adress_select20/1
  adress_select2/1 -> adress_select25/1
  valid_in/1 -> delay1/1, edge_detect10/1(in), edge_detect11/1(in)
  [valid_in] -> Counter5/1
  [valid_in] -> Logical/2
  [valid_in] -> Logical1/2
  [rd_valid] -> Counter6/1
  Counter6/1 -> Slice17/1, Slice16/1
  Slice17/1 -> Delay13/1
  Slice16/1 -> Logical7/1, Inverter5/1
  Logical6/1 -> Delay2/1
  Inverter5/1 -> Logical6/1
  Delay2/1 -> [qdr0_re]
  Logical7/1 -> Delay3/1
  Delay3/1 -> [qdr1_re]
  [rd_valid] -> Logical6/2
  [rd_valid] -> Logical7/2
  Relational1/1 -> edge_detect1/1(in)
  adress_select3/1 -> adress_select19/1
  qdr_latency/1 -> adress_select7/1
  qdr0/2 -> adress_select9/1  "q0dv"
  adress_select4/1 -> adress_select24/1
  qdr_latency1/1 -> adress_select13/1
  qdr1/2 -> adress_select15/1  "q1dv"
  adress_select5/1 -> adress_select23/1
  [qdr0_we] -> adress_select5/2
  delay/1 -> [data_in]
  [data_in] -> adress_select6/1
  [qdr1_we] -> adress_select6/2
  adress_select6/1 -> adress_select28/1
  adress_select7/1 -> adress_select39/1
  adress_select8/1 -> adress_select40/1
  adress_select9/1 -> adress_select41/1
  adress_select10/1 -> adress_select42/1
  adress_select11/1 -> adress_select43/1
  adress_select12/1 -> adress_select44/1
  adress_select13/1 -> adress_select45/1
  adress_select14/1 -> adress_select46/1
  adress_select15/1 -> adress_select47/1
  adress_select16/1 -> adress_select48/1
  adress_select17/1 -> adress_select49/1
  adress_select18/1 -> adress_select50/1
  [qdr0_dv] -> Inverter/1
  Inverter/1 -> Logical2/1
  [qdr1_dv] -> Logical2/2
  Logical2/1 -> Convert/1
  Convert/1 -> [qdr_select]
  [qdr0_dv] -> Logical3/1
  [qdr1_dv] -> Logical3/2
  Logical3/1 -> [buffer_we]
  [buffer_wr_adress] -> Delay7/1
  Delay7/1 -> buffer/1
  [buffer_wr_adress] -> Delay8/1
  Delay8/1 -> buffer1/1
  [buffer_wr_adress] -> Delay15/1
  [buffer_wr_adress] -> Delay16/1
  Delay15/1 -> buffer2/1
  Delay16/1 -> buffer3/1
  Counter4/1 -> Slice6/1, Slice5/1, Slice7/1, Slice2/1
  [buffer_re] -> Counter4/1
  Concat2/1 -> [buffer_rd_adress]
  Slice6/1 -> Concat2/1
  Slice5/1 -> Concat2/2
  [buffer_select] -> Delay17/1
  Delay17/1 -> Mux8/1, Mux9/1
  Delay1/1 -> edge_detect2/1(in)
  edge_detect2/1(out) -> sync_out/1
  Delay18/1 -> out0/1
  Delay19/1 -> valid0/1
  Delay20/1 -> valid1/1
  Delay21/1 -> out1/1
  [op_valid] -> Delay22/1
  Delay22/1 -> Delay23/1, Delay14/1
  Delay23/1 -> Delay20/1
  [buffer_we] -> qdr_latency2/1
  qdr_latency2/1 -> [buffer_re]
  Slice7/1 -> Inverter3/1
  Logical8/1 -> [op_valid]
  Inverter3/1 -> Logical8/1
  [buffer_re] -> Logical8/2
  Slice18/1 -> buffer/2, [din_buffer0]
  Delay14/1 -> Delay1/1, Delay1/2, Delay19/1
  Slice2/1 -> [buffer_select]
  Constant2/1 -> Relational1/1
  [valid_in_end] -> Counter7/1, Counter21/2
  Counter7/1 -> Relational1/2
  Relational2/1 -> edge_detect6/1(in)
  Constant3/1 -> Relational2/1
  Convert2/1 -> [rd_valid]
  Counter8/1 -> Convert2/1
  Logical4/1 -> [rd_start]
  edge_detect6/1(out) -> Logical4/1
  edge_detect1/1(out) -> Logical5/1
  Logical5/1 -> [rd_end]
  [rd_end] -> Counter8/1
  [rd_start] -> Counter8/2
  Delay13/1 -> [rd_address0], [rd_address1]
  Counter2/1 -> Slice1/1, Slice3/1, Slice4/1
  Slice4/1 -> Concat1/1
  Slice1/1 -> Concat1/2
  Slice3/1 -> Concat1/3
  Concat1/1 -> [buffer_wr_adress]
  [buffer_we] -> Counter2/1
  Counter1/1 -> Relational2/2
  delay1/1 -> [valid_in]
  edge_detect10/1(out) -> [valid_in_start]
  edge_detect11/1(out) -> [valid_in_end]
  [valid_in_start] -> Counter1/1, Counter20/2
  Counter20/1 -> Convert3/1
  [rd_start] -> Counter20/1
  Convert3/1 -> Logical4/2
  Counter21/1 -> Convert5/1
  [rd_end] -> Counter21/1
  Convert5/1 -> Logical5/2
  delay2/1 -> delay/1
  adress_select19/1 -> adress_select29/1
  adress_select20/1 -> adress_select30/1
  adress_select21/1 -> adress_select31/1
  adress_select22/1 -> adress_select32/1
  adress_select23/1 -> adress_select33/1
  adress_select24/1 -> adress_select34/1
  adress_select25/1 -> adress_select35/1
  adress_select26/1 -> adress_select36/1
  adress_select27/1 -> adress_select37/1
  adress_select28/1 -> adress_select38/1
  adress_select29/1 -> qdr0/1, qdr_latency/1  "q0r"
  adress_select30/1 -> qdr0/2  "q0w"
  adress_select31/1 -> qdr0/3
  adress_select32/1 -> qdr0/4  "q0a"
  adress_select33/1 -> qdr0/5  "q0din"
  adress_select34/1 -> qdr1/1, qdr_latency1/1  "q1r"
  adress_select35/1 -> qdr1/2  "q1w"
  adress_select36/1 -> qdr1/3
  adress_select37/1 -> qdr1/4  "q1a"
  adress_select38/1 -> qdr1/5  "q1din"
  adress_select39/1 -> [qdr0_dv]
  adress_select40/1 -> [qdr0_dout]
  adress_select41/1 -> Terminator2/1
  adress_select42/1 -> Terminator1/1
  adress_select43/1 -> phy_ready0/1
  adress_select44/1 -> cal_fail0/1
  adress_select45/1 -> [qdr1_dv]
  adress_select46/1 -> [qdr1_dout]
  adress_select47/1 -> Terminator3/1
  adress_select48/1 -> Terminator5/1
  adress_select49/1 -> phy_ready1/1
  adress_select50/1 -> cal_fail1/1

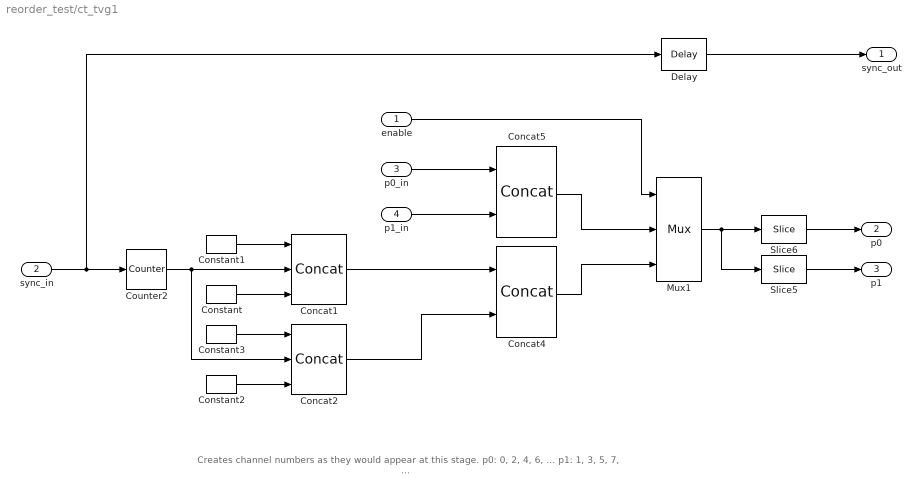
== system reorder_test/ct_tvg1 ==
  note: Creates channel numbers as they would appear at this stage.
      | p0: 0, 2, 4, 6, ...
      | p1: 1, 3, 5, 7, ...
  enable : Inport
  sync_in : Inport  Port=2
  p0_in : Inport  Port=3
  p1_in : Inport  Port=4
  Concat1 : xbsIndex_r4/Concat  num_inputs=3  dbl_ovrd=off  block_type=concat
  Concat2 : xbsIndex_r4/Concat  num_inputs=3  dbl_ovrd=off  block_type=concat
  Concat4 : xbsIndex_r4/Concat  num_inputs=2  dbl_ovrd=off  block_type=concat
  Concat5 : xbsIndex_r4/Concat  num_inputs=2  dbl_ovrd=off  block_type=concat
  Constant : xbsIndex_r4/Constant  const=0  gui_display_data_type=Fixed-point  arith_type=Unsigned  n_bits=1  bin_pt=0  preci_type=Single  exp_width=8  frac_width=24  explicit_period=on  period=1  equ=P=C  opselect=C  inp2=PCIN>>17  opr=+  inp1=P  carry=CIN  dbl_ovrd=off  block_type=constant
      settings: block_version=11.4
  Constant1 : xbsIndex_r4/Constant  const=ant  gui_display_data_type=Fixed-point  arith_type=Unsigned  n_bits=4  bin_pt=0  preci_type=Single  exp_width=8  frac_width=24  explicit_period=on  period=1  equ=P=C  opselect=C  inp2=PCIN>>17  opr=+  inp1=P  carry=CIN  dbl_ovrd=off  block_type=constant
      settings: block_version=11.4
  Constant2 : xbsIndex_r4/Constant  const=1  gui_display_data_type=Fixed-point  arith_type=Unsigned  n_bits=1  bin_pt=0  preci_type=Single  exp_width=8  frac_width=24  explicit_period=on  period=1  equ=P=C  opselect=C  inp2=PCIN>>17  opr=+  inp1=P  carry=CIN  dbl_ovrd=off  block_type=constant
      settings: block_version=11.4
  Constant3 : xbsIndex_r4/Constant  const=ant  gui_display_data_type=Fixed-point  arith_type=Unsigned  n_bits=4  bin_pt=0  preci_type=Single  exp_width=8  frac_width=24  explicit_period=on  period=1  equ=P=C  opselect=C  inp2=PCIN>>17  opr=+  inp1=P  carry=CIN  dbl_ovrd=off  block_type=constant
      settings: block_version=11.4
  Counter2 : xbsIndex_r4/Counter  cnt_type=Free Running  cnt_to=10  operation=Up  start_count=0  cnt_by_val=1  arith_type=Unsigned  n_bits=num_channels_bits - 1  bin_pt=0  load_pin=off  rst=on  en=off  explicit_period=on  period=1  dbl_ovrd=off  use_behavioral_HDL=off  implementation=Fabric  block_type=counter
      settings: block_version=11.4
  Delay : xbsIndex_r4/Delay  rst=off  infoeditControl=Selection of Reset will increase slice count due to use of real FFs and instead of SRLs  en=off  latency=1  dbl_ovrd=off  reg_retiming=on  block_type=delay
      settings: block_version=11.4
  Mux1 : xbsIndex_r4/Mux  inputs=2  en=off  latency=1  precision=Full  arith_type=Unsigned  n_bits=16  bin_pt=14  quantization=Truncate  overflow=Wrap  dbl_ovrd=off  block_type=mux
      settings: block_version=11.4
  Slice5 : xbsIndex_r4/Slice  nbits=channel_bits * 2  boolean_output=off  mode=Lower Bit Location + Width  bit1=0  base1=MSB of Input  bit0=0  base0=LSB of Input  dbl_ovrd=off  block_type=slice
      settings: block_version=10.1.3
  Slice6 : xbsIndex_r4/Slice  nbits=channel_bits * 2  boolean_output=off  mode=Lower Bit Location + Width  bit1=0  base1=MSB of Input  bit0=channel_bits * 2  base0=LSB of Input  dbl_ovrd=off  block_type=slice
      settings: block_version=10.1.3
  sync_out : Outport
  p0 : Outport  Port=2
  p1 : Outport  Port=3
  wires:
  Concat2/1 -> Concat4/2
  Concat1/1 -> Concat4/1
  Constant3/1 -> Concat2/1
  Constant2/1 -> Concat2/3
  Constant1/1 -> Concat1/1
  Constant/1 -> Concat1/3
  Counter2/1 -> Concat2/2, Concat1/2
  sync_in/1 -> Delay/1, Counter2/1
  Delay/1 -> sync_out/1
  p1_in/1 -> Concat5/2
  p0_in/1 -> Concat5/1
  enable/1 -> Mux1/1
  Slice6/1 -> p0/1
  Slice5/1 -> p1/1
  Concat5/1 -> Mux1/2
  Mux1/1 -> Slice6/1, Slice5/1
  Concat4/1 -> Mux1/3
